simulink model "extended_state_observor"  (R2019b)
settings: Solver=FixedStepAuto  StartTime=0.0  StopTime=15  FixedStep=0.001  RelTol=1e-3
settings Model: Creator=henry  LastModifiedBy=henry

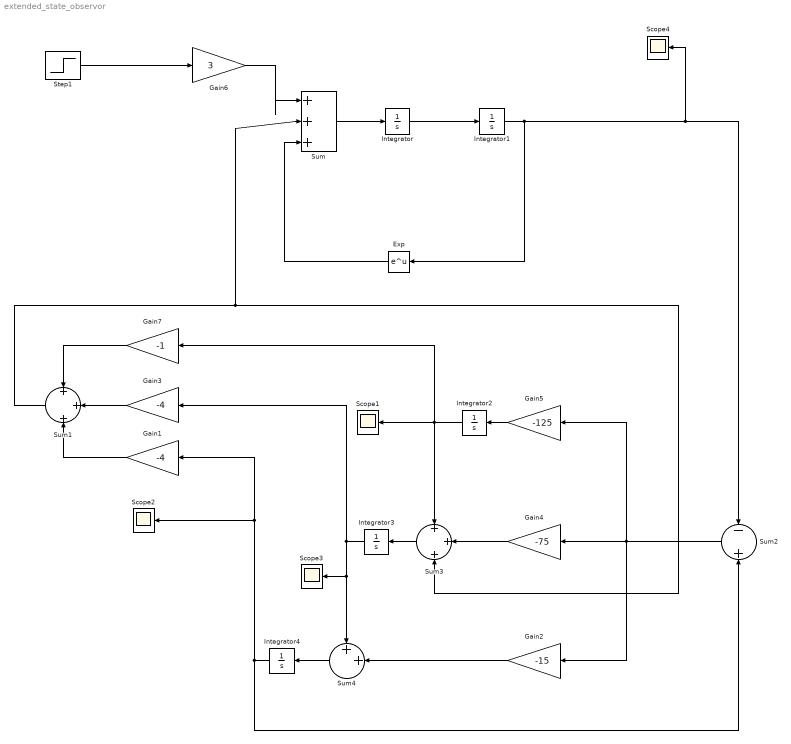
== system extended_state_observor ==
  Exp : Math  SignedPower=off  SaturateOnIntegerOverflow=on
  Gain1 : Gain  Gain=-4
  Gain2 : Gain  Gain=-15
  Gain3 : Gain  Gain=-4
  Gain4 : Gain  Gain=-75
  Gain5 : Gain  Gain=-125
  Gain6 : Gain  Gain=3
  Gain7 : Gain  Gain=-1
  Integrator : Integrator  InitialCondition=-1.5
  Integrator1 : Integrator  InitialCondition=1.75
  Integrator2 : Integrator
  Integrator3 : Integrator
  Integrator4 : Integrator
  Scope{1..4} (4 alike) : Scope
  Step1 : Step  Time=6  SampleTime=0
  Sum : Sum  Inputs=|+++
  Sum1 : Sum  Inputs=+|+|+
  Sum2 : Sum  Inputs=-|+
  Sum3 : Sum  Inputs=+|+|+
  Sum4 : Sum  Inputs=++|
  wires:
  Sum/1 -> Integrator/1
  Sum2/1 -> Gain5/1, Gain2/1, Gain4/1
  Gain2/1 -> Sum4/2
  Gain4/1 -> Sum3/2
  Gain5/1 -> Integrator2/1
  Integrator2/1 -> Gain7/1, Scope1/1, Sum3/1
  Sum3/1 -> Integrator3/1
  Integrator3/1 -> Gain3/1, Scope3/1, Sum4/1
  Sum4/1 -> Integrator4/1
  Integrator4/1 -> Gain1/1, Scope2/1, Sum2/2
  Sum1/1 -> Sum/2, Sum3/3
  Integrator1/1 -> Exp/1, Scope4/1, Sum2/1
  Gain6/1 -> Sum/1
  Step1/1 -> Gain6/1
  Gain7/1 -> Sum1/1
  Gain1/1 -> Sum1/3
  Gain3/1 -> Sum1/2
  Integrator/1 -> Integrator1/1
  Exp/1 -> Sum/3
